simulink model "position_impedance_hold"  (R2021a)
settings: Solver=FixedStepDiscrete  StartTime=0.0  StopTime=inf  FixedStep=0.001  RelTol=1e-3  EnableMultiTasking=on
PreLoadFcn:
  | set_param(gcs, 'RTWSystemTargetFile', 'franka_emika_panda.tlc');
  | % demos_common_configs();
values from neighbouring files (symbols this model uses):
  q_init = [65*pi/128, 59*pi/512, 0, -315 * pi/512, 0, 48*pi/64, 14*pi/64]    [position_impedance_hold_init.m]
libraries: franka_simulink_library x4
settings Model: SimulationMode=external  ExtModeTrigDuration=10000  Creator=vasi_ko  LastModifiedBy=host
settings SolverCC: AlgebraicLoopSolver=TrustRegion
settings DataIOCC: LimitDataPoints=on  SaveFormat=Array  ReturnWorkspaceOutputs=off
settings OptimizationCC: DefaultParameterBehavior=Inlined  EnhancedBackFolding=on  PassReuseOutputArgsThreshold=0  OptimizeBlockOrder=speed  DifferentSizesBufferReuse=on  OptimizationCustomize=off
settings DebuggingCC: SolverPrmCheckMsg=warning  ParameterTunabilityLossMsg=error  SFUnexpectedBacktrackingDiag=warning  SFNoUnconditionalDefaultTransitionDiag=warning  SFExecutionAtInitializationDiag=none  SFMachineParentedDataDiag=warning  ArithmeticOperatorsInVariantConditions=warning
settings HardwareCC: ProdBitPerLong=64  ProdHWDeviceType=Intel->x86-64 (Linux 64)
settings ModelReferenceCC: PropagateSignalLabelsOutOfModel=off
settings SFSimCC: SimUseLocalCustomCode=off  MATLABDynamicMemAlloc=off  CustomCodeUndefinedFunction=UseInterfaceOnly  SimTargetLang=C++
settings RTWCC: Description=Generic Real-Time Target  SystemTargetFile=franka_emika_panda.tlc  RTWVerbose=off  RTWUseLocalCustomCode=off  Toolchain=Franka Simulink | gmake (64-bit linux)  BuildConfiguration=Faster Runs  TargetLang=C++
settings CodeAppCC: ForceParamTrailComments=on  OperatorAnnotations=on
settings STFCustomTargetCC: TargetLangStandard=C99 (ISO)  ModelReferenceCompliant=off  MatFileLogging=on  SystemTargetFile=franka_emika_panda.tlc
settings GRTTargetCC: ModelReferenceCompliant=off  ParMdlRefBuildCompliant=off  CompOptLevelCompliant=off  ConcurrentExecutionCompliant=off  CombineOutputUpdateFcns=off  CPPClassGenCompliant=off  GRTInterface=on  ExtModeStaticAlloc=on  ExtModeTransport=1  ExtModeMexFile=ext_xcp  ExtModeIntrfLevel=Level2 - Open
settings ConfigComp: CovMetricSettings=dw  CovSaveCumulativeToWorkspaceVar=on  CovSaveSingleToWorkspaceVar=on  CovExternalEMLEnable=off  CovSFcnEnable=off

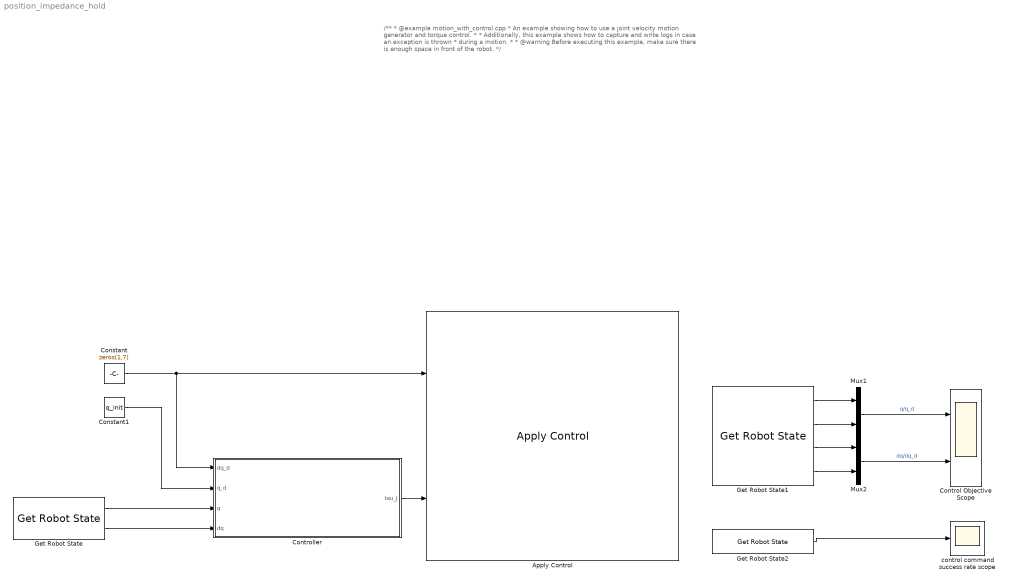
== system position_impedance_hold ==
  note: /**
      |  * @example motion_with_control.cpp
      |  * An example showing how to use a joint velocity motion generator and torque control.
      |  *
      |  * Additionally, this example shows how to capture and write logs in case an exception is thrown
      |  * during a motion.
      |  *
      |  * @warning Before executing this example, make sure there is enough space in front of the robot.
      |  */
  Apply Control : franka_simulink_library/Apply Control  robot_ip=robot_ip  gripper_attached=off  control_mode=Torque Control - Joint Velocities  controller_choice=Joint Impedance Controller  elbow_control=on  collision_thresholds=collision_behavior  joint_impedance=joint_impedance  cartesian_impedance=cartesian_impedance  load_inertia=load_inertia  EE_T_K=EE_T_K  init_joint_configuration_req=off  init_joint_configuration=q_init
      settings: SourceProductName=Franka Emika
  Constant : Constant  Value=zeros(1,7)  VectorParams1D=off
  Constant1 : Constant  Value=q_init  VectorParams1D=off
  Control Objective Scope : Scope  NumInputPorts=2
  Controller : Subsystem
      mask Display:
      | % pos = get_param(gcb, 'Position');
      | 
      | disp('{\bf\fontsize{18}PD Controller}', 'texmode','on');
      | 
      | block_icon('Controller')
      | 
      | port_label('output',1,'tau_J_d');
      | 
      | port_label('input',2,'q_d');
      | port_label('input',1,'dq_d');
      | port_label('input',3,'q');
      | port_label('input',4,'dq');
  Get Robot State : franka_simulink_library/Get Robot State  robot_ip=robot_ip  signals_requested='q dq'
      settings: SourceProductName=Franka Emika
  Get Robot State1 : franka_simulink_library/Get Robot State  robot_ip=robot_ip  signals_requested='q q_d dq dq_d'
      settings: SourceProductName=Franka Emika
  Get Robot State2 : franka_simulink_library/Get Robot State  robot_ip=robot_ip  signals_requested='control_command_success_rate'
      settings: SourceProductName=Franka Emika
  Mux1 : Mux  Inputs=2
  Mux2 : Mux  Inputs=2
  control command success rate scope : Scope
  wires:
  Constant/1 -> Apply Control/1, Controller/1(dq_d)
  Constant1/1 -> Controller/2(q_d)
  Controller/1(tau_J) -> Apply Control/2
  Mux2/1 -> Control Objective Scope/2  "dq/dq_d"
  Get Robot State/2 -> Controller/4(dq)
  Mux1/1 -> Control Objective Scope/1  "q/q_d"
  Get Robot State/1 -> Controller/3(q)
  Get Robot State1/1 -> Mux1/1
  Get Robot State1/2 -> Mux1/2
  Get Robot State1/3 -> Mux2/1
  Get Robot State1/4 -> Mux2/2
  Get Robot State2/1 -> control command success rate scope/1

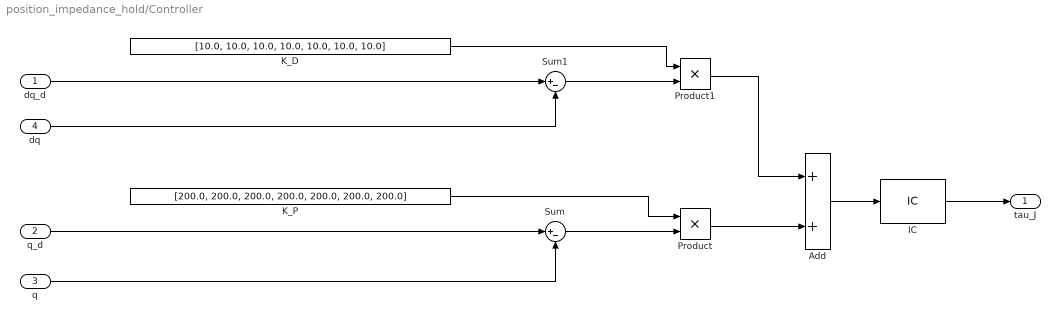
== system position_impedance_hold/Controller ==
  dq_d : Inport
  q_d : Inport  Port=2
  q : Inport  Port=3
  dq : Inport  Port=4
  Add : Sum
  IC : InitialCondition  Value=zeros(1,7)
  K_D : Constant  Value=[10.0, 10.0, 10.0, 10.0, 10.0, 10.0, 10.0]  VectorParams1D=off  SampleTime=-1
  K_P : Constant  Value=[200.0, 200.0, 200.0, 200.0, 200.0, 200.0, 200.0]  VectorParams1D=off  SampleTime=-1
  Product : Product
  Product1 : Product
  Sum : Sum  Inputs=|+-
  Sum1 : Sum  Inputs=|+-
  tau_J : Outport  VectorParamsAs1DForOutWhenUnconnected=off
  wires:
  IC/1 -> tau_J/1
  Add/1 -> IC/1
  Sum1/1 -> Product1/2
  dq/1 -> Sum1/2
  q_d/1 -> Sum/1
  dq_d/1 -> Sum1/1
  Product1/1 -> Add/1
  Product/1 -> Add/2
  K_D/1 -> Product1/1
  K_P/1 -> Product/1
  Sum/1 -> Product/2
  q/1 -> Sum/2
